simulink model "SensorConditioning"  (R2025a)
settings: Solver=FixedStepDiscrete  StartTime=0.0  StopTime=10.0  RelTol=1e-3
settings Model: Creator=mfussi  LastModifiedBy=mfussi
settings OptimizationCC: DefaultParameterBehavior=Inlined  EnhancedBackFolding=on  PassReuseOutputArgsAs=Individual arguments  ZeroExternalMemoryAtStartup=off  ZeroInternalMemoryAtStartup=off  OptimizeBlockOrder=speed  DifferentSizesBufferReuse=on  OptimizationCustomize=off  EfficientTunableParamExpr=on
settings DebuggingCC: ParameterTunabilityLossMsg=error
settings SFSimCC: MATLABDynamicMemAlloc=off
settings RTWCC: SystemTargetFile=ert.tlc  TemplateMakefile=ert_default_tmf  Description=Embedded Coder
settings CodeAppCC: ForceParamTrailComments=on  IgnoreCustomStorageClasses=off  OperatorAnnotations=on  SimulinkDataObjDesc=on  SFDataObjDesc=on  InsertBlockDesc=on
settings ERTTargetCC: ExtModeTransport=0.0  ExtModeStaticAlloc=off  ExtModeMexFile=ext_comm  ExtModeIntrfLevel=Level1  ERTCustomFileTemplate=example_file_process.tlc  TargetLangStandard=C99 (ISO)  GenerateSampleERTMain=on

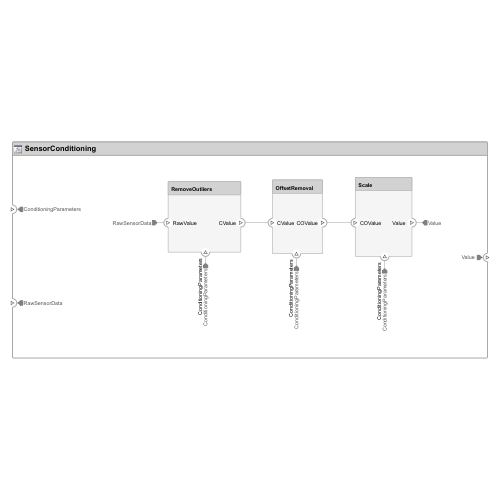
[thumbnail: Simulink's stored preview of the top-level diagram]
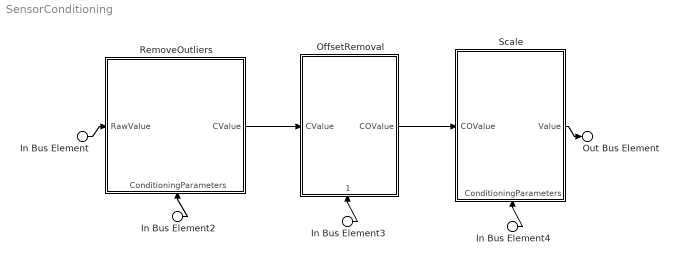
== system SensorConditioning ==
  In Bus Element2 : Inport  PortName=ConditioningParameters
  In Bus Element3 : Inport  PortName=ConditioningParameters
  In Bus Element4 : Inport  PortName=ConditioningParameters
  In Bus Element : Inport  Port=2  PortName=RawSensorData
  OffsetRemoval : Subsystem
      settings: PortSchema="{\"entries\":[{\"content\":{\"headerSize\":26,\"margin\":15,\"minimumSpacing\":25,\"sides\":[{\"content\":{\"connectorIds\":[\"In2\"]},\"type\":\"ConnectorPlacement.EquallySpacedRectSide\",\"uuid\":\"8e6109ac-b489-4864-8b2b-7ebf0beccfe4\"},{\"content\":{\"connectorIds\":[\"Out1\"],\"side\":\"RIGHT\"},\"type\":\"ConnectorPlacement.EquallySpacedRectSide\",\"uuid\":\"71828a7e-6b05-4f57-abc1-6f865453b9f6\"},{\"content\":{\"side\":\"TOP\"},\"type\":\"ConnectorPlacement.EquallySpacedRectSide\",\"uuid\":\"bfeeaaf9-6170-4b48-807f-b679c72692dc\"},{\"content\":{\"connectorIds\":[\"In1\"],\"side\":\"BOTTOM\"},\"type\":\"ConnectorPlacement.EquallySpacedRectSide\",\"uuid\":\"7fbb7351-cb79-4adb-a8e1-9f54598cb7e5\"}]},\"type\":\"ConnectorPlacement.EquallySpacedConnector\",\"uuid\":\"352ed8e9-1880-4bea-97e7-a2aba6f573a0\"}],\"packageUris\":[\"http://schema.mathworks.com/mf0/Connector/R2020b\"],\"version\":\"1.0\"}"
  RemoveOutliers : Subsystem
      settings: PortSchema="{\"entries\":[{\"content\":{\"headerSize\":26,\"margin\":15,\"minimumSpacing\":25,\"sides\":[{\"content\":{\"connectorIds\":[\"In2\"]},\"type\":\"ConnectorPlacement.EquallySpacedRectSide\",\"uuid\":\"8e6109ac-b489-4864-8b2b-7ebf0beccfe4\"},{\"content\":{\"connectorIds\":[\"Out1\"],\"side\":\"RIGHT\"},\"type\":\"ConnectorPlacement.EquallySpacedRectSide\",\"uuid\":\"71828a7e-6b05-4f57-abc1-6f865453b9f6\"},{\"content\":{\"side\":\"TOP\"},\"type\":\"ConnectorPlacement.EquallySpacedRectSide\",\"uuid\":\"bfeeaaf9-6170-4b48-807f-b679c72692dc\"},{\"content\":{\"connectorIds\":[\"In1\"],\"side\":\"BOTTOM\"},\"type\":\"ConnectorPlacement.EquallySpacedRectSide\",\"uuid\":\"a62ede27-fdb3-483d-aea9-721bd3ca17a1\"}]},\"type\":\"ConnectorPlacement.EquallySpacedConnector\",\"uuid\":\"352ed8e9-1880-4bea-97e7-a2aba6f573a0\"}],\"packageUris\":[\"http://schema.mathworks.com/mf0/Connector/R2020b\"],\"version\":\"1.0\"}"
  Scale : Subsystem
      settings: PortSchema="{\"entries\":[{\"content\":{\"headerSize\":26,\"margin\":15,\"minimumSpacing\":25,\"sides\":[{\"content\":{\"connectorIds\":[\"In2\"]},\"type\":\"ConnectorPlacement.EquallySpacedRectSide\",\"uuid\":\"8e6109ac-b489-4864-8b2b-7ebf0beccfe4\"},{\"content\":{\"connectorIds\":[\"Out1\"],\"side\":\"RIGHT\"},\"type\":\"ConnectorPlacement.EquallySpacedRectSide\",\"uuid\":\"71828a7e-6b05-4f57-abc1-6f865453b9f6\"},{\"content\":{\"side\":\"TOP\"},\"type\":\"ConnectorPlacement.EquallySpacedRectSide\",\"uuid\":\"bfeeaaf9-6170-4b48-807f-b679c72692dc\"},{\"content\":{\"connectorIds\":[\"In1\"],\"side\":\"BOTTOM\"},\"type\":\"ConnectorPlacement.EquallySpacedRectSide\",\"uuid\":\"9fdc861f-779b-409b-a4c1-7295406c40af\"}]},\"type\":\"ConnectorPlacement.EquallySpacedConnector\",\"uuid\":\"352ed8e9-1880-4bea-97e7-a2aba6f573a0\"}],\"packageUris\":[\"http://schema.mathworks.com/mf0/Connector/R2020b\"],\"version\":\"1.0\"}"
  Out Bus Element : Outport  PortName=Value
  wires:
  OffsetRemoval/1(COValue) -> Scale/2(COValue)
  RemoveOutliers/1(CValue) -> OffsetRemoval/2(CValue)
  In Bus Element/1 -> RemoveOutliers/2(RawValue)
  Scale/1("Value ") -> Out Bus Element/1
  In Bus Element2/1 -> RemoveOutliers/1(ConditioningParameters)
  In Bus Element3/1 -> OffsetRemoval/1(ConditioningParameters)
  In Bus Element4/1 -> Scale/1(ConditioningParameters)

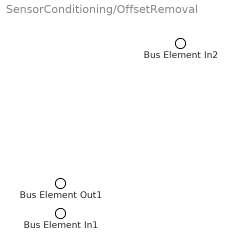
== system SensorConditioning/OffsetRemoval ==
  Bus Element In2 : Inport  PortName=ConditioningParameters
  Bus Element In1 : Inport  Port=2  PortName=CValue
  Bus Element Out1 : Outport  PortName=COValue

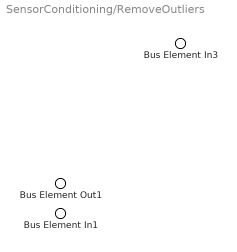
== system SensorConditioning/RemoveOutliers ==
  Bus Element In3 : Inport  PortName=ConditioningParameters
  Bus Element In1 : Inport  Port=2  PortName=RawValue
  Bus Element Out1 : Outport  PortName=CValue

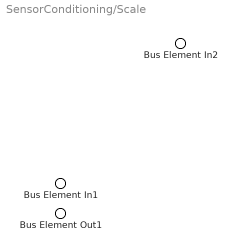
== system SensorConditioning/Scale ==
  Bus Element In2 : Inport  PortName=ConditioningParameters
  Bus Element In1 : Inport  Port=2  PortName=COValue
  Bus Element Out1 : Outport  PortName=Value
